simulink model "model_2"  (R2018b)
settings: Solver=ode4  StartTime=0.0  StopTime=10.0  FixedStep=1e-2  RelTol=1e-3
values from neighbouring files (symbols this model uses):
  A = lambda(i)    [Dyskretny.m]    (also in DyskretnyVsCiagly.m = expm(h*A_c); Kapitalizacja.m = 1.04)
  A_c = [0 1;-I -N]    [DyskretnyVsCiagly.m]
  B = 0    [Dyskretny.m]    (also in DyskretnyVsCiagly.m = double(int(expm(t*A_c)*B_c,t,0,h)); Kapitalizacja.m)
  B_c = [0;1]    [DyskretnyVsCiagly.m]
  C = 1    [Dyskretny.m]    (also in DyskretnyVsCiagly.m = C_c; Kapitalizacja.m)
  C_c = [1 0; 0 1]    [DyskretnyVsCiagly.m]
  D = 0    [Dyskretny.m]    (also in DyskretnyVsCiagly.m = D_c; Kapitalizacja.m)
  D_c = [0;0]    [DyskretnyVsCiagly.m]
  h = 1    [Dyskretny.m]    (also in DyskretnyVsCiagly.m; Kapitalizacja.m = cap_rate)
  Start = 10    [Dyskretny.m]    (also in DyskretnyVsCiagly.m = 5; Kapitalizacja.m = 10000)
  Start_c = Start    (= 5)    [DyskretnyVsCiagly.m]
settings Model: Creator=bion  LastModifiedBy=bion

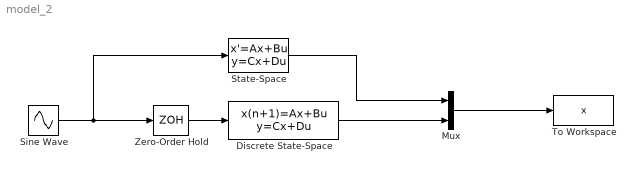
== system model_2 ==
  Discrete State-Space : DiscreteStateSpace  A=A  B=B  C=C  D=D  InitialCondition=Start  SampleTime=h
  Mux : Mux  Inputs=2
  Sine Wave : Sin  SampleTime=0
  State-Space : StateSpace  A=A_c  B=B_c  C=C_c  D=D_c  InitialCondition=Start_c
  To Workspace : ToWorkspace  VariableName=x  SampleTime=1e-2
  Zero-Order Hold : ZeroOrderHold  SampleTime=h
  wires:
  Discrete State-Space/1 -> Mux/2
  Zero-Order Hold/1 -> Discrete State-Space/1
  Sine Wave/1 -> State-Space/1, Zero-Order Hold/1
  State-Space/1 -> Mux/1
  Mux/1 -> To Workspace/1
